simulink library "DAQ_lib_HallPositionTorque"  (R2014b)
settings: Solver=ode45  StartTime=0.0  StopTime=10.0  RelTol=1e-3
undefined symbols (not defined in the file): A_lpf_velocity, ANOMALY_INIT, B1_lpf_velocity, B2_lpf_velocity, Calibration, EnableFT, EncoderAngleLimits, EncoderFiltSys, EncoderThreshold, FTCalibration, GearOffsets, IMUAngleLimits, IMUCommand, IMUThreshold, IMUTorsoOffsets, m_XR17D15x, MAX_ANOMALY, MedullaCommand, MicrostrainFiltSys, MODBUS_TIMEOUT, ResetDAQ, ResetYaw, sample_time, standard, STREAMING_TIMEOUT, TareFT, TorsoCOMOffsets, Ts, TsCAN, TsKVH, UseMicrostrainRate
libraries: xpcethercatlib x207, simulink x53, canmsglib x21, speedgoatlib x13, slrtlib x5, speedgoatlib_IO601 x5, dspswit3 x2, dspmtrx3 x2, xpcseriallib x1, SpeedgoatModified x1
(part 5 of 7)

== system DAQ_lib_HallPositionTorque/DAQ Safety Stops IMU Elmo Amplifiers Position and Torque Control with Hall Sensors/DAQ/EtherCATNetwork/EtherCATRobotMicrostrain/LegElmo_1R/EtherCATSubsystem ==
  Control Word : Inport
  Mode of Operation : Inport  Port=2
  Target Position : Inport  Port=3
  Target Torque : Inport  Port=4
  Max Torque : Inport  Port=5
  EtherCAT PDO Receive : xpcethercatlib/EtherCAT PDO Receive  Priority=2  sig_name=Elmo 3.Inputs.Status word  sig_offset=3360  sig_type=uint16  type_size=16  sig_dim=1  device_id=0  sample_time=0.000500
  EtherCAT PDO Receive1 : xpcethercatlib/EtherCAT PDO Receive  Priority=2  sig_name=Elmo 3.Inputs.Mode of operation display  sig_offset=3376  sig_type=int8  type_size=8  sig_dim=1  device_id=0  sample_time=0.000500
  EtherCAT PDO Receive2 : xpcethercatlib/EtherCAT PDO Receive  Priority=2  sig_name=Elmo 3.Inputs.Torque actual value  sig_offset=3456  sig_type=int16  type_size=16  sig_dim=1  device_id=0  sample_time=0.000500
  EtherCAT PDO Receive3 : xpcethercatlib/EtherCAT PDO Receive  Priority=2  sig_name=Elmo 3.Inputs.Position actual value  sig_offset=3392  sig_type=int32  type_size=32  sig_dim=1  device_id=0  sample_time=0.000500
  EtherCAT PDO Receive4 : xpcethercatlib/EtherCAT PDO Receive  Priority=2  sig_name=Elmo 3.Inputs.Velocity actual value  sig_offset=3424  sig_type=int32  type_size=32  sig_dim=1  device_id=0  sample_time=0.000500
  EtherCAT PDO Transmit : xpcethercatlib/EtherCAT PDO Transmit   Priority=3  sig_name=Elmo 3.Outputs.Control word  sig_offset=3360  sig_type=uint16  type_size=16  sig_dim=1  device_id=0  sample_time=0.000500
  EtherCAT PDO Transmit1 : xpcethercatlib/EtherCAT PDO Transmit   Priority=3  sig_name=Elmo 3.Outputs.Mode of operation  sig_offset=3376  sig_type=int8  type_size=8  sig_dim=1  device_id=0  sample_time=0.000500
  EtherCAT PDO Transmit2 : xpcethercatlib/EtherCAT PDO Transmit   Priority=3  sig_name=Elmo 3.Outputs.Target Position  sig_offset=3424  sig_type=int32  type_size=32  sig_dim=1  device_id=0  sample_time=0.000500
  EtherCAT PDO Transmit3 : xpcethercatlib/EtherCAT PDO Transmit   Priority=3  sig_name=Elmo 3.Outputs.Max. Current  sig_offset=3408  sig_type=uint16  type_size=16  sig_dim=1  device_id=0  sample_time=0.000500
  EtherCAT PDO Transmit4 : xpcethercatlib/EtherCAT PDO Transmit   Priority=3  sig_name=Elmo 3.Outputs.Target Torque  sig_offset=3392  sig_type=int16  type_size=16  sig_dim=1  device_id=0  sample_time=0.000500
  Status Word : Outport
  Mode of Operation Display : Outport  Port=2
  Actual Position : Outport  Port=3
  Actual Velocity : Outport  Port=4
  Actual Torque : Outport  Port=5
  wires:
  Max Torque/1 -> EtherCAT PDO Transmit3/1
  EtherCAT PDO Receive/1 -> Status Word/1
  EtherCAT PDO Receive1/1 -> Mode of Operation Display/1
  Mode of Operation/1 -> EtherCAT PDO Transmit1/1
  EtherCAT PDO Receive3/1 -> Actual Position/1
  EtherCAT PDO Receive4/1 -> Actual Velocity/1
  Target Position/1 -> EtherCAT PDO Transmit2/1
  EtherCAT PDO Receive2/1 -> Actual Torque/1
  Control Word/1 -> EtherCAT PDO Transmit/1
  Target Torque/1 -> EtherCAT PDO Transmit4/1

== system DAQ_lib_HallPositionTorque/DAQ Safety Stops IMU Elmo Amplifiers Position and Torque Control with Hall Sensors/DAQ/EtherCATNetwork/EtherCATRobotMicrostrain/LegElmo_1R/Subsystem1 ==
  ControlWordIndex : Inport
  EnableControlWord : Subsystem
  FaultReset : Subsystem
  Merge : Merge  Inputs=4
  NothingControlWord : Subsystem
  ShutdownControlWord : Subsystem
  Switch Case : SwitchCase  CaseConditions={1,2,3}
  ControlWord : Outport
  wires:
  NothingControlWord/1(ControlWord) -> Merge/4
  Merge/1 -> ControlWord/1
  Switch Case/1 -> ShutdownControlWord/Action
  ShutdownControlWord/1(ControlWord) -> Merge/1
  Switch Case/4 -> NothingControlWord/Action
  Switch Case/2 -> EnableControlWord/Action
  ControlWordIndex/1 -> Switch Case/1
  EnableControlWord/1(ControlWord) -> Merge/2
  Switch Case/3 -> FaultReset/Action
  FaultReset/1(ControlWord) -> Merge/3

== system DAQ_lib_HallPositionTorque/DAQ Safety Stops IMU Elmo Amplifiers Position and Torque Control with Hall Sensors/DAQ/EtherCATNetwork/EtherCATRobotMicrostrain/LegElmo_1R/Subsystem10 ==
  ActualValue : Inport
  MaxRatedCurrent : Inport  Port=2
  Data Type Conversion6 : DataTypeConversion  OutDataTypeStr=int16
  Fcn : Fcn  Expr=u(1)*1000/u(2)
  Vector Concatenate : Concatenate
  ScaledValue : Outport
  wires:
  ActualValue/1 -> Vector Concatenate/1
  Vector Concatenate/1 -> Fcn/1
  MaxRatedCurrent/1 -> Vector Concatenate/2
  Data Type Conversion6/1 -> ScaledValue/1
  Fcn/1 -> Data Type Conversion6/1

== system DAQ_lib_HallPositionTorque/DAQ Safety Stops IMU Elmo Amplifiers Position and Torque Control with Hall Sensors/DAQ/EtherCATNetwork/EtherCATRobotMicrostrain/LegElmo_1R/Subsystem2 ==
  StatusWord : Inport
  Bitwise Operator : simulink/Logic and Bit Operations/Bitwise Operator  logicop=AND  UseBitMask=on  BitMask=bin2dec('0000000001001111')  BitMaskRealWorld=Stored Integer
  Compare To Constant : simulink/Logic and Bit Operations/Compare To Constant  relop===  const=bin2dec('0000000001000000')  OutDataTypeStr=boolean
  SwitchOnDisabledMode : Outport
  wires:
  StatusWord/1 -> Bitwise Operator/1
  Compare To Constant/1 -> SwitchOnDisabledMode/1
  Bitwise Operator/1 -> Compare To Constant/1

== system DAQ_lib_HallPositionTorque/DAQ Safety Stops IMU Elmo Amplifiers Position and Torque Control with Hall Sensors/DAQ/EtherCATNetwork/EtherCATRobotMicrostrain/LegElmo_1R/Subsystem3 ==
  StatusWord : Inport
  Bitwise Operator : simulink/Logic and Bit Operations/Bitwise Operator  logicop=AND  UseBitMask=on  BitMask=bin2dec('0000000001101111')  BitMaskRealWorld=Stored Integer
  Compare To Constant : simulink/Logic and Bit Operations/Compare To Constant  relop===  const=bin2dec('0000000000100111')  OutDataTypeStr=boolean
  EnabledMode : Outport
  wires:
  StatusWord/1 -> Bitwise Operator/1
  Compare To Constant/1 -> EnabledMode/1
  Bitwise Operator/1 -> Compare To Constant/1

== system DAQ_lib_HallPositionTorque/DAQ Safety Stops IMU Elmo Amplifiers Position and Torque Control with Hall Sensors/DAQ/EtherCATNetwork/EtherCATRobotMicrostrain/LegElmo_1R/Subsystem4 ==
  StatusWord : Inport
  Bitwise Operator : simulink/Logic and Bit Operations/Bitwise Operator  logicop=AND  UseBitMask=on  BitMask=bin2dec('0000000001101111')  BitMaskRealWorld=Stored Integer
  Compare To Constant : simulink/Logic and Bit Operations/Compare To Constant  relop===  const=bin2dec('0000000000100001')  OutDataTypeStr=boolean
  ReadyToSwitchOnMode : Outport
  wires:
  StatusWord/1 -> Bitwise Operator/1
  Compare To Constant/1 -> ReadyToSwitchOnMode/1
  Bitwise Operator/1 -> Compare To Constant/1

== system DAQ_lib_HallPositionTorque/DAQ Safety Stops IMU Elmo Amplifiers Position and Torque Control with Hall Sensors/DAQ/EtherCATNetwork/EtherCATRobotMicrostrain/LegElmo_1R/Subsystem5 ==
  StatusWord : Inport
  Bitwise Operator : simulink/Logic and Bit Operations/Bitwise Operator  logicop=AND  UseBitMask=on  BitMask=bin2dec('0000000000001000')  BitMaskRealWorld=Stored Integer
  Compare To Constant : simulink/Logic and Bit Operations/Compare To Constant  relop===  const=bin2dec('0000000000001000')  OutDataTypeStr=boolean
  FaultMode : Outport
  wires:
  StatusWord/1 -> Bitwise Operator/1
  Compare To Constant/1 -> FaultMode/1
  Bitwise Operator/1 -> Compare To Constant/1

== system DAQ_lib_HallPositionTorque/DAQ Safety Stops IMU Elmo Amplifiers Position and Torque Control with Hall Sensors/DAQ/EtherCATNetwork/EtherCATRobotMicrostrain/LegElmo_1R/Subsystem6 ==
  ScaledValue : Inport
  MaxRatedCurrent : Inport  Port=2
  Fcn : Fcn  Expr=u(1)*u(2)/1000
  Vector Concatenate : Concatenate
  ActualValue : Outport
  wires:
  ScaledValue/1 -> Vector Concatenate/1
  Vector Concatenate/1 -> Fcn/1
  MaxRatedCurrent/1 -> Vector Concatenate/2
  Fcn/1 -> ActualValue/1

== system DAQ_lib_HallPositionTorque/DAQ Safety Stops IMU Elmo Amplifiers Position and Torque Control with Hall Sensors/DAQ/EtherCATNetwork/EtherCATRobotMicrostrain/LegElmo_1R/Subsystem7 ==
  ActualValue : Inport
  MaxRatedCurrent : Inport  Port=2
  Data Type Conversion6 : DataTypeConversion  OutDataTypeStr=uint16
  Fcn : Fcn  Expr=u(1)*1000/u(2)
  Vector Concatenate : Concatenate
  ScaledValue : Outport
  wires:
  ActualValue/1 -> Vector Concatenate/1
  Vector Concatenate/1 -> Fcn/1
  MaxRatedCurrent/1 -> Vector Concatenate/2
  Data Type Conversion6/1 -> ScaledValue/1
  Fcn/1 -> Data Type Conversion6/1

== system DAQ_lib_HallPositionTorque/DAQ Safety Stops IMU Elmo Amplifiers Position and Torque Control with Hall Sensors/DAQ/EtherCATNetwork/EtherCATRobotMicrostrain/LegElmo_2L/EtherCATSubsystem ==
  Control Word : Inport
  Mode of Operation : Inport  Port=2
  Target Position : Inport  Port=3
  Target Torque : Inport  Port=4
  Max Torque : Inport  Port=5
  EtherCAT PDO Receive : xpcethercatlib/EtherCAT PDO Receive  Priority=2  sig_name=Elmo 4.Inputs.Status word  sig_offset=3248  sig_type=uint16  type_size=16  sig_dim=1  device_id=0  sample_time=0.000500
  EtherCAT PDO Receive1 : xpcethercatlib/EtherCAT PDO Receive  Priority=2  sig_name=Elmo 4.Inputs.Mode of operation display  sig_offset=3264  sig_type=int8  type_size=8  sig_dim=1  device_id=0  sample_time=0.000500
  EtherCAT PDO Receive2 : xpcethercatlib/EtherCAT PDO Receive  Priority=2  sig_name=Elmo 4.Inputs.Torque actual value  sig_offset=3344  sig_type=int16  type_size=16  sig_dim=1  device_id=0  sample_time=0.000500
  EtherCAT PDO Receive3 : xpcethercatlib/EtherCAT PDO Receive  Priority=2  sig_name=Elmo 4.Inputs.Position actual value  sig_offset=3280  sig_type=int32  type_size=32  sig_dim=1  device_id=0  sample_time=0.000500
  EtherCAT PDO Receive4 : xpcethercatlib/EtherCAT PDO Receive  Priority=2  sig_name=Elmo 4.Inputs.Velocity actual value  sig_offset=3312  sig_type=int32  type_size=32  sig_dim=1  device_id=0  sample_time=0.000500
  EtherCAT PDO Transmit : xpcethercatlib/EtherCAT PDO Transmit   Priority=3  sig_name=Elmo 4.Outputs.Control word  sig_offset=3248  sig_type=uint16  type_size=16  sig_dim=1  device_id=0  sample_time=0.000500
  EtherCAT PDO Transmit1 : xpcethercatlib/EtherCAT PDO Transmit   Priority=3  sig_name=Elmo 4.Outputs.Mode of operation  sig_offset=3264  sig_type=int8  type_size=8  sig_dim=1  device_id=0  sample_time=0.000500
  EtherCAT PDO Transmit2 : xpcethercatlib/EtherCAT PDO Transmit   Priority=3  sig_name=Elmo 4.Outputs.Target Position  sig_offset=3312  sig_type=int32  type_size=32  sig_dim=1  device_id=0  sample_time=0.000500
  EtherCAT PDO Transmit3 : xpcethercatlib/EtherCAT PDO Transmit   Priority=3  sig_name=Elmo 4.Outputs.Max. Current  sig_offset=3296  sig_type=uint16  type_size=16  sig_dim=1  device_id=0  sample_time=0.000500
  EtherCAT PDO Transmit4 : xpcethercatlib/EtherCAT PDO Transmit   Priority=3  sig_name=Elmo 4.Outputs.Target Torque  sig_offset=3280  sig_type=int16  type_size=16  sig_dim=1  device_id=0  sample_time=0.000500
  Status Word : Outport
  Mode of Operation Display : Outport  Port=2
  Actual Position : Outport  Port=3
  Actual Velocity : Outport  Port=4
  Actual Torque : Outport  Port=5
  wires:
  Max Torque/1 -> EtherCAT PDO Transmit3/1
  EtherCAT PDO Receive/1 -> Status Word/1
  EtherCAT PDO Receive1/1 -> Mode of Operation Display/1
  Mode of Operation/1 -> EtherCAT PDO Transmit1/1
  EtherCAT PDO Receive3/1 -> Actual Position/1
  EtherCAT PDO Receive4/1 -> Actual Velocity/1
  Target Position/1 -> EtherCAT PDO Transmit2/1
  EtherCAT PDO Receive2/1 -> Actual Torque/1
  Control Word/1 -> EtherCAT PDO Transmit/1
  Target Torque/1 -> EtherCAT PDO Transmit4/1

== system DAQ_lib_HallPositionTorque/DAQ Safety Stops IMU Elmo Amplifiers Position and Torque Control with Hall Sensors/DAQ/EtherCATNetwork/EtherCATRobotMicrostrain/LegElmo_2L/Subsystem1 ==
  ControlWordIndex : Inport
  EnableControlWord : Subsystem
  FaultReset : Subsystem
  Merge : Merge  Inputs=4
  NothingControlWord : Subsystem
  ShutdownControlWord : Subsystem
  Switch Case : SwitchCase  CaseConditions={1,2,3}
  ControlWord : Outport
  wires:
  NothingControlWord/1(ControlWord) -> Merge/4
  Merge/1 -> ControlWord/1
  Switch Case/1 -> ShutdownControlWord/Action
  ShutdownControlWord/1(ControlWord) -> Merge/1
  Switch Case/4 -> NothingControlWord/Action
  Switch Case/2 -> EnableControlWord/Action
  ControlWordIndex/1 -> Switch Case/1
  EnableControlWord/1(ControlWord) -> Merge/2
  Switch Case/3 -> FaultReset/Action
  FaultReset/1(ControlWord) -> Merge/3

== system DAQ_lib_HallPositionTorque/DAQ Safety Stops IMU Elmo Amplifiers Position and Torque Control with Hall Sensors/DAQ/EtherCATNetwork/EtherCATRobotMicrostrain/LegElmo_2L/Subsystem10 ==
  ActualValue : Inport
  MaxRatedCurrent : Inport  Port=2
  Data Type Conversion6 : DataTypeConversion  OutDataTypeStr=int16
  Fcn : Fcn  Expr=u(1)*1000/u(2)
  Vector Concatenate : Concatenate
  ScaledValue : Outport
  wires:
  ActualValue/1 -> Vector Concatenate/1
  Vector Concatenate/1 -> Fcn/1
  MaxRatedCurrent/1 -> Vector Concatenate/2
  Data Type Conversion6/1 -> ScaledValue/1
  Fcn/1 -> Data Type Conversion6/1

== system DAQ_lib_HallPositionTorque/DAQ Safety Stops IMU Elmo Amplifiers Position and Torque Control with Hall Sensors/DAQ/EtherCATNetwork/EtherCATRobotMicrostrain/LegElmo_2L/Subsystem2 ==
  StatusWord : Inport
  Bitwise Operator : simulink/Logic and Bit Operations/Bitwise Operator  logicop=AND  UseBitMask=on  BitMask=bin2dec('0000000001001111')  BitMaskRealWorld=Stored Integer
  Compare To Constant : simulink/Logic and Bit Operations/Compare To Constant  relop===  const=bin2dec('0000000001000000')  OutDataTypeStr=boolean
  SwitchOnDisabledMode : Outport
  wires:
  StatusWord/1 -> Bitwise Operator/1
  Compare To Constant/1 -> SwitchOnDisabledMode/1
  Bitwise Operator/1 -> Compare To Constant/1

== system DAQ_lib_HallPositionTorque/DAQ Safety Stops IMU Elmo Amplifiers Position and Torque Control with Hall Sensors/DAQ/EtherCATNetwork/EtherCATRobotMicrostrain/LegElmo_2L/Subsystem3 ==
  StatusWord : Inport
  Bitwise Operator : simulink/Logic and Bit Operations/Bitwise Operator  logicop=AND  UseBitMask=on  BitMask=bin2dec('0000000001101111')  BitMaskRealWorld=Stored Integer
  Compare To Constant : simulink/Logic and Bit Operations/Compare To Constant  relop===  const=bin2dec('0000000000100111')  OutDataTypeStr=boolean
  EnabledMode : Outport
  wires:
  StatusWord/1 -> Bitwise Operator/1
  Compare To Constant/1 -> EnabledMode/1
  Bitwise Operator/1 -> Compare To Constant/1

== system DAQ_lib_HallPositionTorque/DAQ Safety Stops IMU Elmo Amplifiers Position and Torque Control with Hall Sensors/DAQ/EtherCATNetwork/EtherCATRobotMicrostrain/LegElmo_2L/Subsystem4 ==
  StatusWord : Inport
  Bitwise Operator : simulink/Logic and Bit Operations/Bitwise Operator  logicop=AND  UseBitMask=on  BitMask=bin2dec('0000000001101111')  BitMaskRealWorld=Stored Integer
  Compare To Constant : simulink/Logic and Bit Operations/Compare To Constant  relop===  const=bin2dec('0000000000100001')  OutDataTypeStr=boolean
  ReadyToSwitchOnMode : Outport
  wires:
  StatusWord/1 -> Bitwise Operator/1
  Compare To Constant/1 -> ReadyToSwitchOnMode/1
  Bitwise Operator/1 -> Compare To Constant/1

== system DAQ_lib_HallPositionTorque/DAQ Safety Stops IMU Elmo Amplifiers Position and Torque Control with Hall Sensors/DAQ/EtherCATNetwork/EtherCATRobotMicrostrain/LegElmo_2L/Subsystem5 ==
  StatusWord : Inport
  Bitwise Operator : simulink/Logic and Bit Operations/Bitwise Operator  logicop=AND  UseBitMask=on  BitMask=bin2dec('0000000000001000')  BitMaskRealWorld=Stored Integer
  Compare To Constant : simulink/Logic and Bit Operations/Compare To Constant  relop===  const=bin2dec('0000000000001000')  OutDataTypeStr=boolean
  FaultMode : Outport
  wires:
  StatusWord/1 -> Bitwise Operator/1
  Compare To Constant/1 -> FaultMode/1
  Bitwise Operator/1 -> Compare To Constant/1

== system DAQ_lib_HallPositionTorque/DAQ Safety Stops IMU Elmo Amplifiers Position and Torque Control with Hall Sensors/DAQ/EtherCATNetwork/EtherCATRobotMicrostrain/LegElmo_2L/Subsystem6 ==
  ScaledValue : Inport
  MaxRatedCurrent : Inport  Port=2
  Fcn : Fcn  Expr=u(1)*u(2)/1000
  Vector Concatenate : Concatenate
  ActualValue : Outport
  wires:
  ScaledValue/1 -> Vector Concatenate/1
  Vector Concatenate/1 -> Fcn/1
  MaxRatedCurrent/1 -> Vector Concatenate/2
  Fcn/1 -> ActualValue/1

== system DAQ_lib_HallPositionTorque/DAQ Safety Stops IMU Elmo Amplifiers Position and Torque Control with Hall Sensors/DAQ/EtherCATNetwork/EtherCATRobotMicrostrain/LegElmo_2L/Subsystem7 ==
  ActualValue : Inport
  MaxRatedCurrent : Inport  Port=2
  Data Type Conversion6 : DataTypeConversion  OutDataTypeStr=uint16
  Fcn : Fcn  Expr=u(1)*1000/u(2)
  Vector Concatenate : Concatenate
  ScaledValue : Outport
  wires:
  ActualValue/1 -> Vector Concatenate/1
  Vector Concatenate/1 -> Fcn/1
  MaxRatedCurrent/1 -> Vector Concatenate/2
  Data Type Conversion6/1 -> ScaledValue/1
  Fcn/1 -> Data Type Conversion6/1

== system DAQ_lib_HallPositionTorque/DAQ Safety Stops IMU Elmo Amplifiers Position and Torque Control with Hall Sensors/DAQ/EtherCATNetwork/EtherCATRobotMicrostrain/LegElmo_2R/EtherCATSubsystem ==
  Control Word : Inport
  Mode of Operation : Inport  Port=2
  Target Position : Inport  Port=3
  Target Torque : Inport  Port=4
  Max Torque : Inport  Port=5
  EtherCAT PDO Receive : xpcethercatlib/EtherCAT PDO Receive  Priority=2  sig_name=Elmo 2.Inputs.Status word  sig_offset=3472  sig_type=uint16  type_size=16  sig_dim=1  device_id=0  sample_time=0.000500
  EtherCAT PDO Receive1 : xpcethercatlib/EtherCAT PDO Receive  Priority=2  sig_name=Elmo 2.Inputs.Mode of operation display  sig_offset=3488  sig_type=int8  type_size=8  sig_dim=1  device_id=0  sample_time=0.000500
  EtherCAT PDO Receive2 : xpcethercatlib/EtherCAT PDO Receive  Priority=2  sig_name=Elmo 2.Inputs.Torque actual value  sig_offset=3568  sig_type=int16  type_size=16  sig_dim=1  device_id=0  sample_time=0.000500
  EtherCAT PDO Receive3 : xpcethercatlib/EtherCAT PDO Receive  Priority=2  sig_name=Elmo 2.Inputs.Position actual value  sig_offset=3504  sig_type=int32  type_size=32  sig_dim=1  device_id=0  sample_time=0.000500
  EtherCAT PDO Receive4 : xpcethercatlib/EtherCAT PDO Receive  Priority=2  sig_name=Elmo 2.Inputs.Velocity actual value  sig_offset=3536  sig_type=int32  type_size=32  sig_dim=1  device_id=0  sample_time=0.000500
  EtherCAT PDO Transmit : xpcethercatlib/EtherCAT PDO Transmit   Priority=3  sig_name=Elmo 2.Outputs.Control word  sig_offset=3472  sig_type=uint16  type_size=16  sig_dim=1  device_id=0  sample_time=0.000500
  EtherCAT PDO Transmit1 : xpcethercatlib/EtherCAT PDO Transmit   Priority=3  sig_name=Elmo 2.Outputs.Mode of operation  sig_offset=3488  sig_type=int8  type_size=8  sig_dim=1  device_id=0  sample_time=0.000500
  EtherCAT PDO Transmit2 : xpcethercatlib/EtherCAT PDO Transmit   Priority=3  sig_name=Elmo 2.Outputs.Target Position  sig_offset=3536  sig_type=int32  type_size=32  sig_dim=1  device_id=0  sample_time=0.000500
  EtherCAT PDO Transmit3 : xpcethercatlib/EtherCAT PDO Transmit   Priority=3  sig_name=Elmo 2.Outputs.Max. Current  sig_offset=3520  sig_type=uint16  type_size=16  sig_dim=1  device_id=0  sample_time=0.000500
  EtherCAT PDO Transmit4 : xpcethercatlib/EtherCAT PDO Transmit   Priority=3  sig_name=Elmo 2.Outputs.Target Torque  sig_offset=3504  sig_type=int16  type_size=16  sig_dim=1  device_id=0  sample_time=0.000500
  Status Word : Outport
  Mode of Operation Display : Outport  Port=2
  Actual Position : Outport  Port=3
  Actual Velocity : Outport  Port=4
  Actual Torque : Outport  Port=5
  wires:
  Max Torque/1 -> EtherCAT PDO Transmit3/1
  EtherCAT PDO Receive/1 -> Status Word/1
  EtherCAT PDO Receive1/1 -> Mode of Operation Display/1
  Mode of Operation/1 -> EtherCAT PDO Transmit1/1
  EtherCAT PDO Receive3/1 -> Actual Position/1
  EtherCAT PDO Receive4/1 -> Actual Velocity/1
  Target Position/1 -> EtherCAT PDO Transmit2/1
  EtherCAT PDO Receive2/1 -> Actual Torque/1
  Control Word/1 -> EtherCAT PDO Transmit/1
  Target Torque/1 -> EtherCAT PDO Transmit4/1

== system DAQ_lib_HallPositionTorque/DAQ Safety Stops IMU Elmo Amplifiers Position and Torque Control with Hall Sensors/DAQ/EtherCATNetwork/EtherCATRobotMicrostrain/LegElmo_2R/Subsystem1 ==
  ControlWordIndex : Inport
  EnableControlWord : Subsystem
  FaultReset : Subsystem
  Merge : Merge  Inputs=4
  NothingControlWord : Subsystem
  ShutdownControlWord : Subsystem
  Switch Case : SwitchCase  CaseConditions={1,2,3}
  ControlWord : Outport
  wires:
  NothingControlWord/1(ControlWord) -> Merge/4
  Merge/1 -> ControlWord/1
  Switch Case/1 -> ShutdownControlWord/Action
  ShutdownControlWord/1(ControlWord) -> Merge/1
  Switch Case/4 -> NothingControlWord/Action
  Switch Case/2 -> EnableControlWord/Action
  ControlWordIndex/1 -> Switch Case/1
  EnableControlWord/1(ControlWord) -> Merge/2
  Switch Case/3 -> FaultReset/Action
  FaultReset/1(ControlWord) -> Merge/3

== system DAQ_lib_HallPositionTorque/DAQ Safety Stops IMU Elmo Amplifiers Position and Torque Control with Hall Sensors/DAQ/EtherCATNetwork/EtherCATRobotMicrostrain/LegElmo_2R/Subsystem10 ==
  ActualValue : Inport
  MaxRatedCurrent : Inport  Port=2
  Data Type Conversion6 : DataTypeConversion  OutDataTypeStr=int16
  Fcn : Fcn  Expr=u(1)*1000/u(2)
  Vector Concatenate : Concatenate
  ScaledValue : Outport
  wires:
  ActualValue/1 -> Vector Concatenate/1
  Vector Concatenate/1 -> Fcn/1
  MaxRatedCurrent/1 -> Vector Concatenate/2
  Data Type Conversion6/1 -> ScaledValue/1
  Fcn/1 -> Data Type Conversion6/1

== system DAQ_lib_HallPositionTorque/DAQ Safety Stops IMU Elmo Amplifiers Position and Torque Control with Hall Sensors/DAQ/EtherCATNetwork/EtherCATRobotMicrostrain/LegElmo_2R/Subsystem2 ==
  StatusWord : Inport
  Bitwise Operator : simulink/Logic and Bit Operations/Bitwise Operator  logicop=AND  UseBitMask=on  BitMask=bin2dec('0000000001001111')  BitMaskRealWorld=Stored Integer
  Compare To Constant : simulink/Logic and Bit Operations/Compare To Constant  relop===  const=bin2dec('0000000001000000')  OutDataTypeStr=boolean
  SwitchOnDisabledMode : Outport
  wires:
  StatusWord/1 -> Bitwise Operator/1
  Compare To Constant/1 -> SwitchOnDisabledMode/1
  Bitwise Operator/1 -> Compare To Constant/1

== system DAQ_lib_HallPositionTorque/DAQ Safety Stops IMU Elmo Amplifiers Position and Torque Control with Hall Sensors/DAQ/EtherCATNetwork/EtherCATRobotMicrostrain/LegElmo_2R/Subsystem3 ==
  StatusWord : Inport
  Bitwise Operator : simulink/Logic and Bit Operations/Bitwise Operator  logicop=AND  UseBitMask=on  BitMask=bin2dec('0000000001101111')  BitMaskRealWorld=Stored Integer
  Compare To Constant : simulink/Logic and Bit Operations/Compare To Constant  relop===  const=bin2dec('0000000000100111')  OutDataTypeStr=boolean
  EnabledMode : Outport
  wires:
  StatusWord/1 -> Bitwise Operator/1
  Compare To Constant/1 -> EnabledMode/1
  Bitwise Operator/1 -> Compare To Constant/1

== system DAQ_lib_HallPositionTorque/DAQ Safety Stops IMU Elmo Amplifiers Position and Torque Control with Hall Sensors/DAQ/EtherCATNetwork/EtherCATRobotMicrostrain/LegElmo_2R/Subsystem4 ==
  StatusWord : Inport
  Bitwise Operator : simulink/Logic and Bit Operations/Bitwise Operator  logicop=AND  UseBitMask=on  BitMask=bin2dec('0000000001101111')  BitMaskRealWorld=Stored Integer
  Compare To Constant : simulink/Logic and Bit Operations/Compare To Constant  relop===  const=bin2dec('0000000000100001')  OutDataTypeStr=boolean
  ReadyToSwitchOnMode : Outport
  wires:
  StatusWord/1 -> Bitwise Operator/1
  Compare To Constant/1 -> ReadyToSwitchOnMode/1
  Bitwise Operator/1 -> Compare To Constant/1

== system DAQ_lib_HallPositionTorque/DAQ Safety Stops IMU Elmo Amplifiers Position and Torque Control with Hall Sensors/DAQ/EtherCATNetwork/EtherCATRobotMicrostrain/LegElmo_2R/Subsystem5 ==
  StatusWord : Inport
  Bitwise Operator : simulink/Logic and Bit Operations/Bitwise Operator  logicop=AND  UseBitMask=on  BitMask=bin2dec('0000000000001000')  BitMaskRealWorld=Stored Integer
  Compare To Constant : simulink/Logic and Bit Operations/Compare To Constant  relop===  const=bin2dec('0000000000001000')  OutDataTypeStr=boolean
  FaultMode : Outport
  wires:
  StatusWord/1 -> Bitwise Operator/1
  Compare To Constant/1 -> FaultMode/1
  Bitwise Operator/1 -> Compare To Constant/1

== system DAQ_lib_HallPositionTorque/DAQ Safety Stops IMU Elmo Amplifiers Position and Torque Control with Hall Sensors/DAQ/EtherCATNetwork/EtherCATRobotMicrostrain/LegElmo_2R/Subsystem6 ==
  ScaledValue : Inport
  MaxRatedCurrent : Inport  Port=2
  Fcn : Fcn  Expr=u(1)*u(2)/1000
  Vector Concatenate : Concatenate
  ActualValue : Outport
  wires:
  ScaledValue/1 -> Vector Concatenate/1
  Vector Concatenate/1 -> Fcn/1
  MaxRatedCurrent/1 -> Vector Concatenate/2
  Fcn/1 -> ActualValue/1

== system DAQ_lib_HallPositionTorque/DAQ Safety Stops IMU Elmo Amplifiers Position and Torque Control with Hall Sensors/DAQ/EtherCATNetwork/EtherCATRobotMicrostrain/LegElmo_2R/Subsystem7 ==
  ActualValue : Inport
  MaxRatedCurrent : Inport  Port=2
  Data Type Conversion6 : DataTypeConversion  OutDataTypeStr=uint16
  Fcn : Fcn  Expr=u(1)*1000/u(2)
  Vector Concatenate : Concatenate
  ScaledValue : Outport
  wires:
  ActualValue/1 -> Vector Concatenate/1
  Vector Concatenate/1 -> Fcn/1
  MaxRatedCurrent/1 -> Vector Concatenate/2
  Data Type Conversion6/1 -> ScaledValue/1
  Fcn/1 -> Data Type Conversion6/1

== system DAQ_lib_HallPositionTorque/DAQ Safety Stops IMU Elmo Amplifiers Position and Torque Control with Hall Sensors/DAQ/SerialInterfaces/FTCAN/CANMessageOut/ReadFirmwareVersion ==
  Action Port : ActionPort
  CAN Pack : canmsglib/CAN Pack  MsgList=(none)  MsgName=ReadFirmwareVersion  MsgIDType=Standard (11-bit identifier)  MsgIdentifier=hex2dec('20F')  MsgLength=0  NSignals=0  StartBits=0  SignalSizes=0  ByteOrders=0  DataTypes=0  MultiplexTypes=0  MultiplexValues=0  Factors=0  Offsets=0  Minimums=0  Maximums=0  Remote=off
      settings: DataFormat=manually specified signals
  Constant : Constant  Value=0  SampleTime=TsCAN
  CanMessage : Outport
  wires:
  CAN Pack/1 -> CanMessage/1
  Constant/1 -> CAN Pack/1

== system DAQ_lib_HallPositionTorque/DAQ Safety Stops IMU Elmo Amplifiers Position and Torque Control with Hall Sensors/DAQ/SerialInterfaces/FTCAN/CANMessageOut/ReadMatrixRow1 ==
  Action Port : ActionPort
  CAN Pack : canmsglib/CAN Pack  MsgList=(none)  MsgName=ReadMatrix  MsgIDType=Standard (11-bit identifier)  MsgIdentifier=hex2dec('202')  MsgLength=1  SignalInfo=AxisRow$0$8$1$2$1$0$1$0$-Inf$Inf$#  NSignals=1  StartBits=str2num('[int32(0)]')  SignalSizes=str2num('[int32(8)]')  ByteOrders=str2num('[int32(1)]')  DataTypes=str2num('[int32(2)]')  MultiplexTypes=str2num('[int32(1)]')  MultiplexValues=str2num('[double(0)]')  Factors=str2num('[double(1)]')  Offsets=str2num('[double(0)]')  Minimums=str2num('[double(-Inf)]')  Maximums=str2num('[double(Inf)]')  Remote=off
      settings: DataFormat=manually specified signals
  Constant : Constant  Value=0  SampleTime=TsCAN
  CanMessage : Outport
  wires:
  CAN Pack/1 -> CanMessage/1
  Constant/1 -> CAN Pack/1

== system DAQ_lib_HallPositionTorque/DAQ Safety Stops IMU Elmo Amplifiers Position and Torque Control with Hall Sensors/DAQ/SerialInterfaces/FTCAN/CANMessageOut/ReadMatrixRow2 ==
  Action Port : ActionPort
  CAN Pack : canmsglib/CAN Pack  MsgList=(none)  MsgName=ReadMatrix  MsgIDType=Standard (11-bit identifier)  MsgIdentifier=hex2dec('202')  MsgLength=1  SignalInfo=AxisRow$0$8$1$2$1$0$1$0$-Inf$Inf$#  NSignals=1  StartBits=str2num('[int32(0)]')  SignalSizes=str2num('[int32(8)]')  ByteOrders=str2num('[int32(1)]')  DataTypes=str2num('[int32(2)]')  MultiplexTypes=str2num('[int32(1)]')  MultiplexValues=str2num('[double(0)]')  Factors=str2num('[double(1)]')  Offsets=str2num('[double(0)]')  Minimums=str2num('[double(-Inf)]')  Maximums=str2num('[double(Inf)]')  Remote=off
      settings: DataFormat=manually specified signals
  Constant : Constant  SampleTime=TsCAN
  CanMessage : Outport
  wires:
  CAN Pack/1 -> CanMessage/1
  Constant/1 -> CAN Pack/1

== system DAQ_lib_HallPositionTorque/DAQ Safety Stops IMU Elmo Amplifiers Position and Torque Control with Hall Sensors/DAQ/SerialInterfaces/FTCAN/CANMessageOut/ReadMatrixRow3 ==
  Action Port : ActionPort
  CAN Pack : canmsglib/CAN Pack  MsgList=(none)  MsgName=ReadMatrix  MsgIDType=Standard (11-bit identifier)  MsgIdentifier=hex2dec('202')  MsgLength=1  SignalInfo=AxisRow$0$8$1$2$1$0$1$0$-Inf$Inf$#  NSignals=1  StartBits=str2num('[int32(0)]')  SignalSizes=str2num('[int32(8)]')  ByteOrders=str2num('[int32(1)]')  DataTypes=str2num('[int32(2)]')  MultiplexTypes=str2num('[int32(1)]')  MultiplexValues=str2num('[double(0)]')  Factors=str2num('[double(1)]')  Offsets=str2num('[double(0)]')  Minimums=str2num('[double(-Inf)]')  Maximums=str2num('[double(Inf)]')  Remote=off
      settings: DataFormat=manually specified signals
  Constant : Constant  Value=2  SampleTime=TsCAN
  CanMessage : Outport
  wires:
  CAN Pack/1 -> CanMessage/1
  Constant/1 -> CAN Pack/1

== system DAQ_lib_HallPositionTorque/DAQ Safety Stops IMU Elmo Amplifiers Position and Torque Control with Hall Sensors/DAQ/SerialInterfaces/FTCAN/CANMessageOut/ReadMatrixRow4 ==
  Action Port : ActionPort
  CAN Pack : canmsglib/CAN Pack  MsgList=(none)  MsgName=ReadMatrix  MsgIDType=Standard (11-bit identifier)  MsgIdentifier=hex2dec('202')  MsgLength=1  SignalInfo=AxisRow$0$8$1$2$1$0$1$0$-Inf$Inf$#  NSignals=1  StartBits=str2num('[int32(0)]')  SignalSizes=str2num('[int32(8)]')  ByteOrders=str2num('[int32(1)]')  DataTypes=str2num('[int32(2)]')  MultiplexTypes=str2num('[int32(1)]')  MultiplexValues=str2num('[double(0)]')  Factors=str2num('[double(1)]')  Offsets=str2num('[double(0)]')  Minimums=str2num('[double(-Inf)]')  Maximums=str2num('[double(Inf)]')  Remote=off
      settings: DataFormat=manually specified signals
  Constant : Constant  Value=3  SampleTime=TsCAN
  CanMessage : Outport
  wires:
  CAN Pack/1 -> CanMessage/1
  Constant/1 -> CAN Pack/1

== system DAQ_lib_HallPositionTorque/DAQ Safety Stops IMU Elmo Amplifiers Position and Torque Control with Hall Sensors/DAQ/SerialInterfaces/FTCAN/CANMessageOut/ReadMatrixRow5 ==
  Action Port : ActionPort
  CAN Pack : canmsglib/CAN Pack  MsgList=(none)  MsgName=ReadMatrix  MsgIDType=Standard (11-bit identifier)  MsgIdentifier=hex2dec('202')  MsgLength=1  SignalInfo=AxisRow$0$8$1$2$1$0$1$0$-Inf$Inf$#  NSignals=1  StartBits=str2num('[int32(0)]')  SignalSizes=str2num('[int32(8)]')  ByteOrders=str2num('[int32(1)]')  DataTypes=str2num('[int32(2)]')  MultiplexTypes=str2num('[int32(1)]')  MultiplexValues=str2num('[double(0)]')  Factors=str2num('[double(1)]')  Offsets=str2num('[double(0)]')  Minimums=str2num('[double(-Inf)]')  Maximums=str2num('[double(Inf)]')  Remote=off
      settings: DataFormat=manually specified signals
  Constant : Constant  Value=4  SampleTime=TsCAN
  CanMessage : Outport
  wires:
  CAN Pack/1 -> CanMessage/1
  Constant/1 -> CAN Pack/1

== system DAQ_lib_HallPositionTorque/DAQ Safety Stops IMU Elmo Amplifiers Position and Torque Control with Hall Sensors/DAQ/SerialInterfaces/FTCAN/CANMessageOut/ReadMatrixRow6 ==
  Action Port : ActionPort
  CAN Pack : canmsglib/CAN Pack  MsgList=(none)  MsgName=ReadMatrix  MsgIDType=Standard (11-bit identifier)  MsgIdentifier=hex2dec('202')  MsgLength=1  SignalInfo=AxisRow$0$8$1$2$1$0$1$0$-Inf$Inf$#  NSignals=1  StartBits=str2num('[int32(0)]')  SignalSizes=str2num('[int32(8)]')  ByteOrders=str2num('[int32(1)]')  DataTypes=str2num('[int32(2)]')  MultiplexTypes=str2num('[int32(1)]')  MultiplexValues=str2num('[double(0)]')  Factors=str2num('[double(1)]')  Offsets=str2num('[double(0)]')  Minimums=str2num('[double(-Inf)]')  Maximums=str2num('[double(Inf)]')  Remote=off
      settings: DataFormat=manually specified signals
  Constant : Constant  Value=5  SampleTime=TsCAN
  CanMessage : Outport
  wires:
  CAN Pack/1 -> CanMessage/1
  Constant/1 -> CAN Pack/1

== system DAQ_lib_HallPositionTorque/DAQ Safety Stops IMU Elmo Amplifiers Position and Torque Control with Hall Sensors/DAQ/SerialInterfaces/FTCAN/CANMessageOut/ReadSGData ==
  Action Port : ActionPort
  CAN Pack : canmsglib/CAN Pack  MsgList=(none)  MsgName=ReadFTSerialNumber  MsgIDType=Standard (11-bit identifier)  MsgIdentifier=hex2dec('200')  MsgLength=0  NSignals=0  StartBits=0  SignalSizes=0  ByteOrders=0  DataTypes=0  MultiplexTypes=0  MultiplexValues=0  Factors=0  Offsets=0  Minimums=0  Maximums=0  Remote=off
      settings: DataFormat=manually specified signals
  Constant : Constant  Value=0  SampleTime=TsCAN
  CanMessage : Outport
  wires:
  CAN Pack/1 -> CanMessage/1
  Constant/1 -> CAN Pack/1

== system DAQ_lib_HallPositionTorque/DAQ Safety Stops IMU Elmo Amplifiers Position and Torque Control with Hall Sensors/DAQ/SerialInterfaces/FTCAN/CANMessageOut/SetActiveCalibration ==
  Action Port : ActionPort
  CAN Pack : canmsglib/CAN Pack  MsgList=(none)  MsgName=SetActiveCommand  MsgIDType=Standard (11-bit identifier)  MsgIdentifier=hex2dec('206')  MsgLength=1  SignalInfo=CalibrationIndex$0$8$1$2$1$0$1$0$-Inf$Inf$#  NSignals=1  StartBits=str2num('[int32(0)]')  SignalSizes=str2num('[int32(8)]')  ByteOrders=str2num('[int32(1)]')  DataTypes=str2num('[int32(2)]')  MultiplexTypes=str2num('[int32(1)]')  MultiplexValues=str2num('[double(0)]')  Factors=str2num('[double(1)]')  Offsets=str2num('[double(0)]')  Minimums=str2num('[double(-Inf)]')  Maximums=str2num('[double(Inf)]')  Remote=off
      settings: DataFormat=manually specified signals
  Constant : Constant  Value=0  SampleTime=TsCAN
  CanMessage : Outport
  wires:
  CAN Pack/1 -> CanMessage/1
  Constant/1 -> CAN Pack/1

== system DAQ_lib_HallPositionTorque/DAQ Safety Stops IMU Elmo Amplifiers Position and Torque Control with Hall Sensors/DAQ/SerialInterfaces/FTCAN/ComputeCalibratedTorques/Latch ==
  Gauge : Inport
  Tare : EnablePort
  Bias : Outport  InitialOutput=zeros(6,1,'uint16')
  wires:
  Gauge/1 -> Bias/1

== system DAQ_lib_HallPositionTorque/DAQ Safety Stops IMU Elmo Amplifiers Position and Torque Control with Hall Sensors/DAQ/SerialInterfaces/FTCAN/ComputeCalibratedTorques1/Latch ==
  Gauge : Inport
  Tare : EnablePort
  Bias : Outport  InitialOutput=zeros(6,1,'uint16')
  wires:
  Gauge/1 -> Bias/1

== system DAQ_lib_HallPositionTorque/DAQ Safety Stops IMU Elmo Amplifiers Position and Torque Control with Hall Sensors/DAQ/SerialInterfaces/FTCAN/Read_and_Process_Subsystem/CalibrationMatrixBlock ==
  SGVector : Inport
  ColumnNo : Inport  Port=2
  Enable : EnablePort
  Compare To Constant : simulink/Logic and Bit Operations/Compare To Constant  relop===  const=1  OutDataTypeStr=boolean
  Compare To Constant1 : simulink/Logic and Bit Operations/Compare To Constant  relop===  const=2  OutDataTypeStr=boolean
  Compare To Constant2 : simulink/Logic and Bit Operations/Compare To Constant  relop===  const=3  OutDataTypeStr=boolean
  Compare To Constant3 : simulink/Logic and Bit Operations/Compare To Constant  relop===  const=4  OutDataTypeStr=boolean
  Compare To Constant4 : simulink/Logic and Bit Operations/Compare To Constant  relop===  const=5  OutDataTypeStr=boolean
  Compare To Constant5 : simulink/Logic and Bit Operations/Compare To Constant  relop===  const=6  OutDataTypeStr=boolean
  Fx : Subsystem
  Fy : Subsystem
  Fz : Subsystem
  Matrix Concatenate : Concatenate  NumInputs=6  Mode=Multidimensional array
  Transpose : dspmtrx3/Transpose  Hermitian=off  overflowFlag=off
  Tx : Subsystem
  Ty : Subsystem
  Tz : Subsystem
  CalibrationMatrix : Outport
  wires:
  Compare To Constant/1 -> Fx/Enable
  Compare To Constant1/1 -> Fy/Enable
  Compare To Constant2/1 -> Fz/Enable
  Compare To Constant3/1 -> Tx/Enable
  Compare To Constant4/1 -> Ty/Enable
  Compare To Constant5/1 -> Tz/Enable
  ColumnNo/1 -> Compare To Constant1/1, Compare To Constant5/1, Compare To Constant4/1, Compare To Constant3/1, Compare To Constant2/1, Compare To Constant/1
  Fx/1(Out) -> Matrix Concatenate/1
  Fy/1(Out) -> Matrix Concatenate/2
  Fz/1(Out) -> Matrix Concatenate/3
  Tx/1(Out) -> Matrix Concatenate/4
  Ty/1(Out) -> Matrix Concatenate/5
  Tz/1(Out) -> Matrix Concatenate/6
  Matrix Concatenate/1 -> CalibrationMatrix/1
  SGVector/1 -> Transpose/1
  Transpose/1 -> Tz/1(In), Ty/1(In), Tx/1(In), Fz/1(In), Fy/1(In), Fx/1(In)

== system DAQ_lib_HallPositionTorque/DAQ Safety Stops IMU Elmo Amplifiers Position and Torque Control with Hall Sensors/DAQ/SerialInterfaces/FTCAN/Read_and_Process_Subsystem/CalibrationMatrixBlock1 ==
  SGVector : Inport
  ColumnNo : Inport  Port=2
  Enable : EnablePort
  Compare To Constant : simulink/Logic and Bit Operations/Compare To Constant  relop===  const=1  OutDataTypeStr=boolean
  Compare To Constant1 : simulink/Logic and Bit Operations/Compare To Constant  relop===  const=2  OutDataTypeStr=boolean
  Compare To Constant2 : simulink/Logic and Bit Operations/Compare To Constant  relop===  const=3  OutDataTypeStr=boolean
  Compare To Constant3 : simulink/Logic and Bit Operations/Compare To Constant  relop===  const=4  OutDataTypeStr=boolean
  Compare To Constant4 : simulink/Logic and Bit Operations/Compare To Constant  relop===  const=5  OutDataTypeStr=boolean
  Compare To Constant5 : simulink/Logic and Bit Operations/Compare To Constant  relop===  const=6  OutDataTypeStr=boolean
  Fx : Subsystem
  Fy : Subsystem
  Fz : Subsystem
  Matrix Concatenate : Concatenate  NumInputs=6  Mode=Multidimensional array
  Transpose : dspmtrx3/Transpose  Hermitian=off  overflowFlag=off
  Tx : Subsystem
  Ty : Subsystem
  Tz : Subsystem
  CalibrationMatrix : Outport
  wires:
  Compare To Constant/1 -> Fx/Enable
  Compare To Constant1/1 -> Fy/Enable
  Compare To Constant2/1 -> Fz/Enable
  Compare To Constant3/1 -> Tx/Enable
  Compare To Constant4/1 -> Ty/Enable
  Compare To Constant5/1 -> Tz/Enable
  ColumnNo/1 -> Compare To Constant1/1, Compare To Constant5/1, Compare To Constant4/1, Compare To Constant3/1, Compare To Constant2/1, Compare To Constant/1
  Fx/1(Out) -> Matrix Concatenate/1
  Fy/1(Out) -> Matrix Concatenate/2
  Fz/1(Out) -> Matrix Concatenate/3
  Tx/1(Out) -> Matrix Concatenate/4
  Ty/1(Out) -> Matrix Concatenate/5
  Tz/1(Out) -> Matrix Concatenate/6
  Matrix Concatenate/1 -> CalibrationMatrix/1
  SGVector/1 -> Transpose/1
  Transpose/1 -> Tz/1(In), Ty/1(In), Tx/1(In), Fz/1(In), Fy/1(In), Fx/1(In)

== system DAQ_lib_HallPositionTorque/DAQ Safety Stops IMU Elmo Amplifiers Position and Torque Control with Hall Sensors/DAQ/SerialInterfaces/FTCAN/Read_and_Process_Subsystem/ReadCalibrationMatrixRow_FlipFlops ==
  Reset : Inport
  Status1 : Inport  Port=2
  Status2 : Inport  Port=3
  Status3 : Inport  Port=4
  Logical Operator : Logic  Inputs=3  IconShape=distinctive  AllPortsSameDT=off  OutDataTypeStr=boolean
  Logical Operator1 : Logic  Operator=OR  IconShape=distinctive  AllPortsSameDT=off  OutDataTypeStr=boolean
  Logical Operator2 : Logic  Operator=OR  IconShape=distinctive  AllPortsSameDT=off  OutDataTypeStr=boolean
  Logical Operator3 : Logic  Operator=OR  IconShape=distinctive  AllPortsSameDT=off  OutDataTypeStr=boolean
  Subsystem : Subsystem
  Subsystem1 : Subsystem
  Subsystem2 : Subsystem
  DataRead : Outport
  wires:
  Status1/1 -> Logical Operator1/2, Subsystem/1(Status)
  Reset/1 -> Subsystem2/2(Reset), Logical Operator3/1, Subsystem1/2(Reset), Logical Operator2/1, Subsystem/2(Reset), Logical Operator1/1
  Status2/1 -> Logical Operator2/2, Subsystem1/1(Status)
  Status3/1 -> Logical Operator3/2, Subsystem2/1(Status)
  Subsystem2/1(StatusLatched) -> Logical Operator/3
  Subsystem1/1(StatusLatched) -> Logical Operator/2
  Subsystem/1(StatusLatched) -> Logical Operator/1
  Logical Operator1/1 -> Subsystem/Enable
  Logical Operator2/1 -> Subsystem1/Enable
  Logical Operator3/1 -> Subsystem2/Enable
  Logical Operator/1 -> DataRead/1

== system DAQ_lib_HallPositionTorque/DAQ Safety Stops IMU Elmo Amplifiers Position and Torque Control with Hall Sensors/DAQ/SerialInterfaces/FTCAN/Read_and_Process_Subsystem/ReadCalibrationMatrixRow_FlipFlops1 ==
  Reset : Inport
  Status1 : Inport  Port=2
  Status2 : Inport  Port=3
  Status3 : Inport  Port=4
  Logical Operator : Logic  Inputs=3  IconShape=distinctive  AllPortsSameDT=off  OutDataTypeStr=boolean
  Logical Operator1 : Logic  Operator=OR  IconShape=distinctive  AllPortsSameDT=off  OutDataTypeStr=boolean
  Logical Operator2 : Logic  Operator=OR  IconShape=distinctive  AllPortsSameDT=off  OutDataTypeStr=boolean
  Logical Operator3 : Logic  Operator=OR  IconShape=distinctive  AllPortsSameDT=off  OutDataTypeStr=boolean
  Subsystem : Subsystem
  Subsystem1 : Subsystem
  Subsystem2 : Subsystem
  DataRead : Outport
  wires:
  Status1/1 -> Logical Operator1/2, Subsystem/1(Status)
  Reset/1 -> Subsystem2/2(Reset), Logical Operator3/1, Subsystem1/2(Reset), Logical Operator2/1, Subsystem/2(Reset), Logical Operator1/1
  Status2/1 -> Logical Operator2/2, Subsystem1/1(Status)
  Status3/1 -> Logical Operator3/2, Subsystem2/1(Status)
  Subsystem2/1(StatusLatched) -> Logical Operator/3
  Subsystem1/1(StatusLatched) -> Logical Operator/2
  Subsystem/1(StatusLatched) -> Logical Operator/1
  Logical Operator1/1 -> Subsystem/Enable
  Logical Operator2/1 -> Subsystem1/Enable
  Logical Operator3/1 -> Subsystem2/Enable
  Logical Operator/1 -> DataRead/1

== system DAQ_lib_HallPositionTorque/DAQ Safety Stops IMU Elmo Amplifiers Position and Torque Control with Hall Sensors/DAQ/SerialInterfaces/FTCAN/Read_and_Process_Subsystem/SG_Latch ==
  SG_In : Inport
  Enable : EnablePort
  SG_Out : Outport
  wires:
  SG_In/1 -> SG_Out/1

== system DAQ_lib_HallPositionTorque/DAQ Safety Stops IMU Elmo Amplifiers Position and Torque Control with Hall Sensors/DAQ/SerialInterfaces/FTCAN/Read_and_Process_Subsystem/SG_Latch1 ==
  SG_In : Inport
  Enable : EnablePort
  SG_Out : Outport
  wires:
  SG_In/1 -> SG_Out/1

== system DAQ_lib_HallPositionTorque/DAQ Safety Stops IMU Elmo Amplifiers Position and Torque Control with Hall Sensors/DAQ/SerialInterfaces/FTCAN/Read_and_Process_Subsystem/Select_SetCalibrationMatrixColumn_From_CommandNo ==
  SelectedCommand : Inport
  Merge : Merge  Inputs=6
  ReadRow1 : Subsystem
  ReadRow2 : Subsystem
  ReadRow3 : Subsystem
  ReadRow4 : Subsystem
  ReadRow5 : Subsystem
  ReadRow6 : Subsystem
  Switch Case : SwitchCase  CaseConditions={2,3,4,5,6,7}  ShowDefaultCase=off
  SelectedColumn : Outport
  wires:
  ReadRow1/1(OutValue) -> Merge/1
  Switch Case/1 -> ReadRow1/Action
  Switch Case/6 -> ReadRow6/Action
  Switch Case/5 -> ReadRow5/Action
  Switch Case/4 -> ReadRow4/Action
  Switch Case/3 -> ReadRow3/Action
  Switch Case/2 -> ReadRow2/Action
  ReadRow2/1(OutValue) -> Merge/2
  ReadRow3/1(OutValue) -> Merge/3
  ReadRow4/1(OutValue) -> Merge/4
  ReadRow5/1(OutValue) -> Merge/5
  ReadRow6/1(OutValue) -> Merge/6
  Merge/1 -> SelectedColumn/1
  SelectedCommand/1 -> Switch Case/1

== system DAQ_lib_HallPositionTorque/DAQ Safety Stops IMU Elmo Amplifiers Position and Torque Control with Hall Sensors/DAQ/SerialInterfaces/FTCAN/Read_and_Process_Subsystem/Select_SetCalibrationMatrixColumn_From_CommandNo1 ==
  SelectedCommand : Inport
  Merge : Merge  Inputs=6
  ReadRow1 : Subsystem
  ReadRow2 : Subsystem
  ReadRow3 : Subsystem
  ReadRow4 : Subsystem
  ReadRow5 : Subsystem
  ReadRow6 : Subsystem
  Switch Case : SwitchCase  CaseConditions={2,3,4,5,6,7}  ShowDefaultCase=off
  SelectedColumn : Outport
  wires:
  ReadRow1/1(OutValue) -> Merge/1
  Switch Case/1 -> ReadRow1/Action
  Switch Case/6 -> ReadRow6/Action
  Switch Case/5 -> ReadRow5/Action
  Switch Case/4 -> ReadRow4/Action
  Switch Case/3 -> ReadRow3/Action
  Switch Case/2 -> ReadRow2/Action
  ReadRow2/1(OutValue) -> Merge/2
  ReadRow3/1(OutValue) -> Merge/3
  ReadRow4/1(OutValue) -> Merge/4
  ReadRow5/1(OutValue) -> Merge/5
  ReadRow6/1(OutValue) -> Merge/6
  Merge/1 -> SelectedColumn/1
  SelectedCommand/1 -> Switch Case/1

== system DAQ_lib_HallPositionTorque/DAQ Safety Stops IMU Elmo Amplifiers Position and Torque Control with Hall Sensors/DAQ/SerialInterfaces/FTCAN/Read_and_Process_Subsystem/SelectedIndex_Latch ==
  Enable : EnablePort
  Constant : Constant  OutDataTypeStr=uint8
  SelectedIndexOut : Outport  OutDataTypeStr=uint8  InitialOutput=[0]
  wires:
  Constant/1 -> SelectedIndexOut/1

== system DAQ_lib_HallPositionTorque/DAQ Safety Stops IMU Elmo Amplifiers Position and Torque Control with Hall Sensors/DAQ/SerialInterfaces/FTCAN/Read_and_Process_Subsystem/SelectedIndex_Latch1 ==
  Enable : EnablePort
  Constant : Constant  OutDataTypeStr=uint8
  SelectedIndexOut : Outport  OutDataTypeStr=uint8  InitialOutput=[0]
  wires:
  Constant/1 -> SelectedIndexOut/1

== system DAQ_lib_HallPositionTorque/DAQ Safety Stops IMU Elmo Amplifiers Position and Torque Control with Hall Sensors/DAQ/SerialInterfaces/FTCAN/Read_and_Process_Subsystem/TimestapRecorder ==
  note: Need to make sure that the delay here doesn't cause problems!!!
  TimeIn1 : Inport
  TimeIn2 : Inport  Port=2
  Enable : EnablePort
  TimeOut1 : Outport
  TimeOut2 : Outport  Port=2
  wires:
  TimeIn1/1 -> TimeOut1/1
  TimeIn2/1 -> TimeOut2/1

== system DAQ_lib_HallPositionTorque/DAQ Safety Stops IMU Elmo Amplifiers Position and Torque Control with Hall Sensors/DAQ/SerialInterfaces/FTCAN/Read_and_Process_Subsystem/TimestapRecorder1 ==
  note: Need to make sure that the delay here doesn't cause problems!!!
  TimeIn1 : Inport
  TimeIn2 : Inport  Port=2
  Enable : EnablePort
  TimeOut1 : Outport
  TimeOut2 : Outport  Port=2
  wires:
  TimeIn1/1 -> TimeOut1/1
  TimeIn2/1 -> TimeOut2/1

== system DAQ_lib_HallPositionTorque/DAQ Safety Stops IMU Elmo Amplifiers Position and Torque Control with Hall Sensors/DAQ/SerialInterfaces/FTInterface/Subsystem/ComputeCalibratedTorques ==
  Gauge : Inport
  Cal : Inport  Port=2
  Tare : Inport  Port=3
  ComputeCalibratedTorques : MATLAB Function  TreatAsAtomicUnit=on
  Latch : Subsystem
  Reshape : Reshape
  FT : Outport
  wires:
  Gauge/1 -> Latch/1(Gauge), ComputeCalibratedTorques/1(Gauge)
  ComputeCalibratedTorques/1(FT) -> Reshape/1
  Cal/1 -> ComputeCalibratedTorques/3(Cal)
  Tare/1 -> Latch/Enable
  Reshape/1 -> FT/1
  Latch/1(Bias) -> ComputeCalibratedTorques/2(Bias)

== system DAQ_lib_HallPositionTorque/DAQ Safety Stops IMU Elmo Amplifiers Position and Torque Control with Hall Sensors/DAQ/EtherCATNetwork/EtherCATRobotMicrostrain/LegElmo_1L/Subsystem1/EnableControlWord ==
  Action Port : ActionPort
  Constant : Constant  Value=15  OutDataTypeStr=uint16
  ControlWord : Outport
  wires:
  Constant/1 -> ControlWord/1

== system DAQ_lib_HallPositionTorque/DAQ Safety Stops IMU Elmo Amplifiers Position and Torque Control with Hall Sensors/DAQ/EtherCATNetwork/EtherCATRobotMicrostrain/LegElmo_1L/Subsystem1/FaultReset ==
  Action Port : ActionPort
  Constant : Constant  Value=128  OutDataTypeStr=uint16
  ControlWord : Outport
  wires:
  Constant/1 -> ControlWord/1

== system DAQ_lib_HallPositionTorque/DAQ Safety Stops IMU Elmo Amplifiers Position and Torque Control with Hall Sensors/DAQ/EtherCATNetwork/EtherCATRobotMicrostrain/LegElmo_1L/Subsystem1/NothingControlWord ==
  Action Port : ActionPort
  Constant : Constant  Value=0  OutDataTypeStr=uint16
  ControlWord : Outport
  wires:
  Constant/1 -> ControlWord/1

== system DAQ_lib_HallPositionTorque/DAQ Safety Stops IMU Elmo Amplifiers Position and Torque Control with Hall Sensors/DAQ/EtherCATNetwork/EtherCATRobotMicrostrain/LegElmo_1L/Subsystem1/ShutdownControlWord ==
  Action Port : ActionPort
  Constant : Constant  Value=6  OutDataTypeStr=uint16
  ControlWord : Outport
  wires:
  Constant/1 -> ControlWord/1

== system DAQ_lib_HallPositionTorque/DAQ Safety Stops IMU Elmo Amplifiers Position and Torque Control with Hall Sensors/DAQ/EtherCATNetwork/EtherCATRobotMicrostrain/LegElmo_1R/Subsystem1/EnableControlWord ==
  Action Port : ActionPort
  Constant : Constant  Value=15  OutDataTypeStr=uint16
  ControlWord : Outport
  wires:
  Constant/1 -> ControlWord/1

== system DAQ_lib_HallPositionTorque/DAQ Safety Stops IMU Elmo Amplifiers Position and Torque Control with Hall Sensors/DAQ/EtherCATNetwork/EtherCATRobotMicrostrain/LegElmo_1R/Subsystem1/FaultReset ==
  Action Port : ActionPort
  Constant : Constant  Value=128  OutDataTypeStr=uint16
  ControlWord : Outport
  wires:
  Constant/1 -> ControlWord/1

== system DAQ_lib_HallPositionTorque/DAQ Safety Stops IMU Elmo Amplifiers Position and Torque Control with Hall Sensors/DAQ/EtherCATNetwork/EtherCATRobotMicrostrain/LegElmo_1R/Subsystem1/NothingControlWord ==
  Action Port : ActionPort
  Constant : Constant  Value=0  OutDataTypeStr=uint16
  ControlWord : Outport
  wires:
  Constant/1 -> ControlWord/1
